simulink model "model_2_3"  (R2021b)
settings: Solver=FixedStepAuto  StartTime=0.0  StopTime=5  FixedStep=0.0000005  RelTol=1e-3
settings Model: Creator=den  LastModifiedBy=den

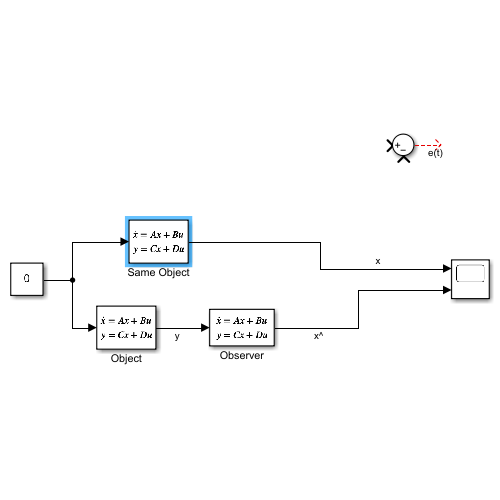
[thumbnail: Simulink's stored preview of the top-level diagram]
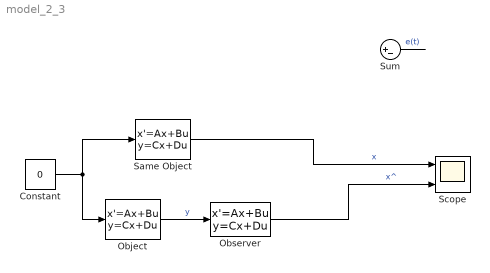
== system model_2_3 ==
  Constant : Constant  Value=0
  Object : StateSpace  A=[0 5 0 0; -5 0 0 0; 0 0 0 1; 0 0 -1 0]  B=[0; 0; 0; 0]  C=[0 9 1 0]  D=0  InitialCondition=[1;1;1;1]
  Observer : StateSpace  A=[0 11/3 -4/27 0; -5 -16/3 -16/27 0; 0 -24 -8/3 1; 0 -42 -17/3 0]  B=[4/27; 16/27; 8/3; 14/3]  C=[1 0 0 0; 0 1 0 0; 0 0 1 0; 0 0 0 1]  D=[0;0;0;0]  InitialCondition=[2;0;0;-1]
  Same Object : StateSpace  A=[0 5 0 0; -5 0 0 0; 0 0 0 1; 0 0 -1 0]  B=[0; 0; 0; 0]  C=[1 0 0 0; 0 1 0 0; 0 0 1 0; 0 0 0 1]  D=[0;0;0;0]  InitialCondition=[1;1;1;1]
  Scope : Scope  NumInputPorts=2
  Sum : Sum  Inputs=|+-
  wires:
  Object/1 -> Observer/1  "y"
  Observer/1 -> Scope/2  "x^"
  Constant/1 -> Same Object/1, Object/1
  Same Object/1 -> Scope/1  "x"
  Sum/1 -> ?  "e(t)"
